simulink model "model2"  (R2018b)
settings: Solver=ode4  StartTime=0.0  StopTime=50.0  FixedStep=0.01  RelTol=1e-3
values from neighbouring files (symbols this model uses):
  c_c = 15000    [dane.m]
  c_w = 200000    [dane.m]
  d_c = 200    [dane.m]
  d_w = 100    [dane.m]
  m_c = 250    [dane.m]
  m_w = 30    [dane.m]
settings Model: Creator=lpa1  LastModifiedBy=lpa1

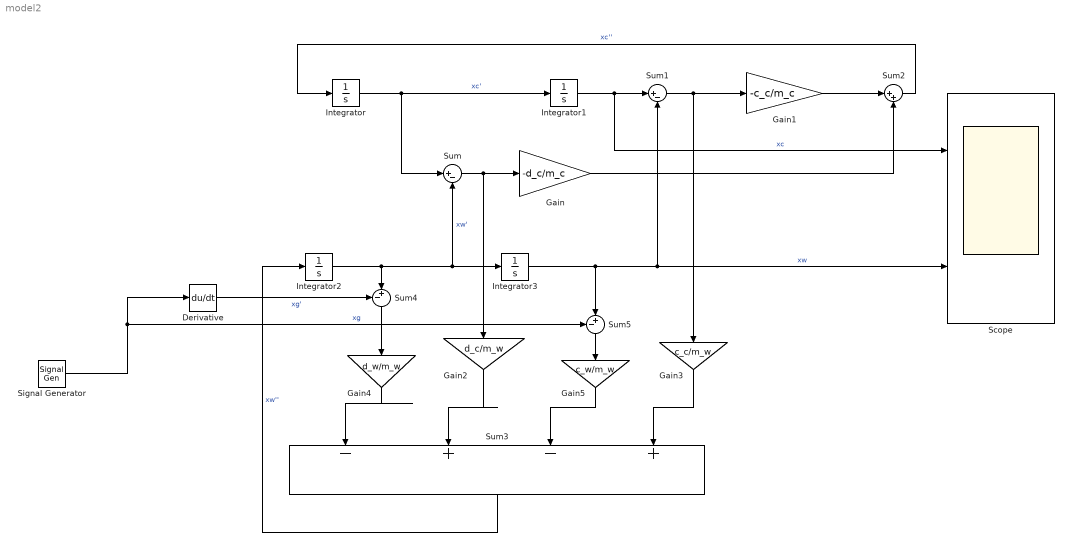
== system model2 ==
  Derivative : Derivative
  Gain : Gain  Gain=-d_c/m_c
  Gain1 : Gain  Gain=-c_c/m_c
  Gain2 : Gain  Gain=d_c/m_w
  Gain3 : Gain  Gain=c_c/m_w
  Gain4 : Gain  Gain=d_w/m_w
  Gain5 : Gain  Gain=c_w/m_w
  Integrator{,1..3} (4 alike) : Integrator
  Scope : Scope  NumInputPorts=2
  Signal Generator : SignalGenerator  WaveForm=square  Amplitude=0.2  Frequency=0.5  Units=rad/sec
  Sum : Sum  Inputs=|+-
  Sum1 : Sum  Inputs=|+-
  Sum2 : Sum  Inputs=|++
  Sum3 : Sum  Inputs=|-+-+
  Sum4 : Sum  Inputs=-+|
  Sum5 : Sum  Inputs=-+|
  wires:
  Integrator/1 -> Sum/1, Integrator1/1  "xc'"
  Integrator2/1 -> Sum4/2, Integrator3/1, Sum/2  "xw'"
  Sum/1 -> Gain/1, Gain2/1
  Integrator1/1 -> Scope/1, Sum1/1  "xc"
  Integrator3/1 -> Scope/2, Sum1/2, Sum5/2  "xw"
  Sum1/1 -> Gain1/1, Gain3/1
  Gain/1 -> Sum2/2
  Gain1/1 -> Sum2/1
  Sum2/1 -> Integrator/1  "xc''"
  Gain4/1 -> Sum3/1
  Gain2/1 -> Sum3/2
  Gain3/1 -> Sum3/4
  Gain5/1 -> Sum3/3
  Sum3/1 -> Integrator2/1  "xw''"
  Signal Generator/1 -> Sum5/1, Derivative/1  "xg"
  Derivative/1 -> Sum4/1  "xg'"
  Sum4/1 -> Gain4/1
  Sum5/1 -> Gain5/1
